simulink model "Aliasing"  (R2017b)
settings: Solver=ode3  StartTime=0.0  StopTime=0.4  RelTol=1e-3
libraries: dspsigops x1
settings Model: Creator=julied  LastModifiedBy=agarwal
settings SolverCC: AutoInsertRateTranBlk=on
settings DataIOCC: LimitDataPoints=on  SaveOutput=off  SignalLogging=off  SaveTime=off
settings OptimizationCC: LifeSpan=inf
settings DebuggingCC: AlgebraicLoopMsg=error  SingleTaskRateTransMsg=error  AllowSymbolicDim=off  SFUnexpectedBacktrackingDiag=warning  SFNoUnconditionalDefaultTransitionDiag=warning  SFExecutionAtInitializationDiag=none
settings CodeAppCC: StateflowObjectComments=on
settings GRTTargetCC: TargetLangStandard=C89/C90 (ANSI)  GeneratePreprocessorConditionals=Disable all

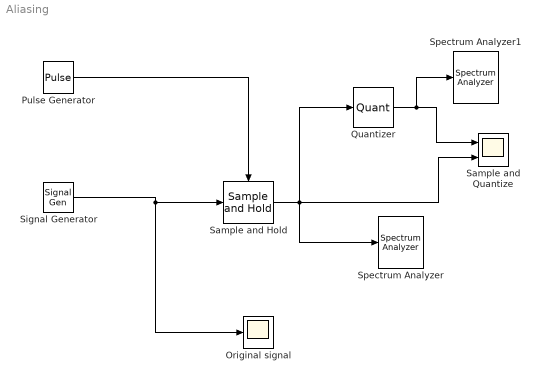
== system Aliasing ==
  Original signal : Scope
  Pulse Generator : DiscretePulseGenerator  PulseType=Time based  Period=1/1000  PulseWidth=50  SampleTime=1/800
  Quantizer : Quantizer  QuantizationInterval=0.1  LinearizeAsGain=off
  Sample and Hold : dspsigops/Sample and Hold  trig=Rising edge  initCond=0  latchinput=off
  Sample and Quantize : Scope  NumInputPorts=2
  Signal Generator : SignalGenerator  Amplitude=5  Frequency=200
  Spectrum Analyzer : SpectrumAnalyzer
  Spectrum Analyzer1 : SpectrumAnalyzer
  wires:
  Pulse Generator/1 -> Sample and Hold/Trigger
  Signal Generator/1 -> Original signal/1, Sample and Hold/1
  Sample and Hold/1 -> Sample and Quantize/2, Quantizer/1, Spectrum Analyzer/1
  Quantizer/1 -> Spectrum Analyzer1/1, Sample and Quantize/1
